simulink model "Power2NoActions"  (Simulink 9.0)
settings: Solver=ode45  StartTime=0.0  StopTime=10.0  RelTol=1e-3  EnableMultiTasking=on
settings Model: SuppressorTable=22 serialization::archive 11 0 6 0 0 0 0 0  Creator=scaife  LastModifiedBy=ktrinh  ExtModeAutoUpdateStatusClock=off
settings DataIOCC: LimitDataPoints=on  SignalLoggingSaveFormat=ModelDataLogs  SignalLoggingName=sigsOut
settings DebuggingCC: SaveWithParameterizedLinksMsg=none  SignalResolutionControl=TryResolveAllWithWarning  MultiTaskDSMMsg=warning  MultiTaskCondExecSysMsg=none  SFUnexpectedBacktrackingDiag=error  SFNoUnconditionalDefaultTransitionDiag=error
settings HardwareCC: TargetUnknown=on
settings SFSimCC: SimParseCustomCode=off
settings GRTTargetCC: CombineOutputUpdateFcns=off  GRTInterface=on

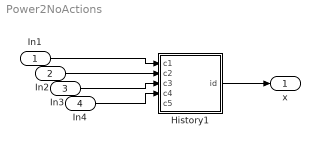
== system Power2NoActions ==
  In1 : Inport  OutDataTypeStr=boolean
  In2 : Inport  Port=2  OutDataTypeStr=boolean
  In3 : Inport  Port=3  OutDataTypeStr=boolean
  In4 : Inport  Port=4  OutDataTypeStr=boolean
  History1 : Stateflow chart  TreatAsAtomicUnit=on
  x : Outport
  wires:
  History1/1(id) -> x/1
  In1/1 -> History1/1(c1)
  In4/1 -> History1/4(c4)
  In3/1 -> History1/3(c3)
  In2/1 -> History1/2(c2)

== stateflow chart History1 ==
  state Power_off
    en: id=0;
  state Power_on
    state Low/
      en: id=1;
    state High/
      en: id=2;
    Power_on -> (history) [order 1] : [c5]
    (default) -> Low
    High -> Low : [c2]
    Low -> High : [c1]
  (default) -> Power_off
  Power_off -> Power_on : [c4]
  Power_on -> Power_off [order 1] : [c3]
  data: c1 input boolean; c2 input boolean; c3 input boolean; c4 input boolean; id output double; c5 input boolean
